simulink model "BallPlate_FLControl"  (R2018b)
settings: Solver=FixedStepAuto  StartTime=0.0  StopTime=20  FixedStep=0.01  RelTol=1e-5
undefined symbols (not defined in the file or in its folder): K
libraries: vrlib x42, simulink x5, aerolibanimutils x3, powerlib_meascontrol x1
(part 2 of 2)

== system BallPlate_FLControl/Feedback linearized 3/Subsystem ==
  tau : Inport
  Ball and Plate dynamic : MATLAB Function  TreatAsAtomicUnit=on
  Constant : Constant  Value=[0.0001;0.0001;.0001;.0001]
  Constant1 : Constant  Value=[.0001;.0001;.0001;.0001]
  Integrator : Integrator  InitialConditionSource=external  InitialCondition=[0;0;0;0]
  Integrator1 : Integrator  InitialConditionSource=external  InitialCondition=[0; 0; 0; 0]
  q : Outport
  dq : Outport  Port=2
  wires:
  tau/1 -> Ball and Plate dynamic/1(tau)
  Integrator1/1 -> q/1, Ball and Plate dynamic/2(q)
  Integrator/1 -> dq/1, Integrator1/1, Ball and Plate dynamic/3(dq)
  Ball and Plate dynamic/1(ddq) -> Integrator/1
  Constant/1 -> Integrator/2
  Constant1/1 -> Integrator1/2

== system BallPlate_FLControl/Feedback linearized 4/Feedback Linearization ==
  nu : Inport
  q : Inport  Port=2
  dq : Inport  Port=3
  Einv_matrix : MATLAB Function  TreatAsAtomicUnit=on
  Gamma_matrix : MATLAB Function  TreatAsAtomicUnit=on
  Matrix Multiply : Product  Multiplication=Matrix(*)
  Matrix Multiply1 : Product  Multiplication=Matrix(*)
  Sum : Sum  Inputs=+-
  u : Outport
  wires:
  Sum/1 -> u/1
  Matrix Multiply1/1 -> Sum/2
  Matrix Multiply/1 -> Sum/1
  Gamma_matrix/1(Gamma) -> Matrix Multiply1/2
  nu/1 -> Matrix Multiply/2
  Einv_matrix/1(Einv) -> Matrix Multiply/1, Matrix Multiply1/1
  dq/1 -> Einv_matrix/2(dq), Gamma_matrix/2(dq)
  q/1 -> Einv_matrix/1(q), Gamma_matrix/1(q)

== system BallPlate_FLControl/Feedback linearized 4/Subsystem ==
  tau : Inport
  Ball and Plate dynamic : MATLAB Function  TreatAsAtomicUnit=on
  Constant : Constant  Value=[0.0001;0.0001;.0001;.0001]
  Constant1 : Constant  Value=[.0001;.0001;.0001;.0001]
  Integrator : Integrator  InitialConditionSource=external  InitialCondition=[0;0;0;0]
  Integrator1 : Integrator  InitialConditionSource=external  InitialCondition=[0; 0; 0; 0]
  q : Outport
  dq : Outport  Port=2
  wires:
  Constant1/1 -> Integrator1/2
  Constant/1 -> Integrator/2
  Ball and Plate dynamic/1(ddq) -> Integrator/1
  Integrator/1 -> Ball and Plate dynamic/3(dq), Integrator1/1, dq/1
  Integrator1/1 -> Ball and Plate dynamic/2(q), q/1
  tau/1 -> Ball and Plate dynamic/1(tau)

== system BallPlate_FLControl/Feedback linearized 5/Feedback Linearization ==
  nu : Inport
  q : Inport  Port=2
  dq : Inport  Port=3
  Einv_matrix : MATLAB Function  TreatAsAtomicUnit=on
  Gamma_matrix : MATLAB Function  TreatAsAtomicUnit=on
  Matrix Multiply : Product  Multiplication=Matrix(*)
  Matrix Multiply1 : Product  Multiplication=Matrix(*)
  Sum : Sum  Inputs=+-
  u : Outport
  wires:
  q/1 -> Gamma_matrix/1(q), Einv_matrix/1(q)
  dq/1 -> Gamma_matrix/2(dq), Einv_matrix/2(dq)
  Einv_matrix/1(Einv) -> Matrix Multiply1/1, Matrix Multiply/1
  nu/1 -> Matrix Multiply/2
  Gamma_matrix/1(Gamma) -> Matrix Multiply1/2
  Matrix Multiply/1 -> Sum/1
  Matrix Multiply1/1 -> Sum/2
  Sum/1 -> u/1

== system BallPlate_FLControl/Feedback linearized 5/Subsystem ==
  tau : Inport
  Ball and Plate dynamic : MATLAB Function  TreatAsAtomicUnit=on
  Constant : Constant  Value=[0.0001;0.0001;.0001;.0001]
  Constant1 : Constant  Value=[.0001;.0001;.0001;.0001]
  Integrator : Integrator  InitialConditionSource=external  InitialCondition=[0;0;0;0]
  Integrator1 : Integrator  InitialConditionSource=external  InitialCondition=[0; 0; 0; 0]
  q : Outport
  dq : Outport  Port=2
  wires:
  tau/1 -> Ball and Plate dynamic/1(tau)
  Integrator1/1 -> q/1, Ball and Plate dynamic/2(q)
  Integrator/1 -> dq/1, Integrator1/1, Ball and Plate dynamic/3(dq)
  Ball and Plate dynamic/1(ddq) -> Integrator/1
  Constant/1 -> Integrator/2
  Constant1/1 -> Integrator1/2

== system BallPlate_FLControl/Visualization parsing1/Rotation composition 1 ==
  alpha : Inport
  beta : Inport  Port=2
  Rotation : MATLAB Function  TreatAsAtomicUnit=on
  Rotation Matrix to VRML Rotation : vrlib/Utilities/Rotation Matrix to VRML Rotation  maxzero=1e-12
      settings: SourceProductName=Simulink 3D Animation  SourceProductBaseCode=VR
  Axis/angle : Outport
  wires:
  alpha/1 -> Rotation/1(alpha)
  Rotation Matrix to VRML Rotation/1 -> Axis/angle/1
  beta/1 -> Rotation/2(beta)
  Rotation/1(R) -> Rotation Matrix to VRML Rotation/1

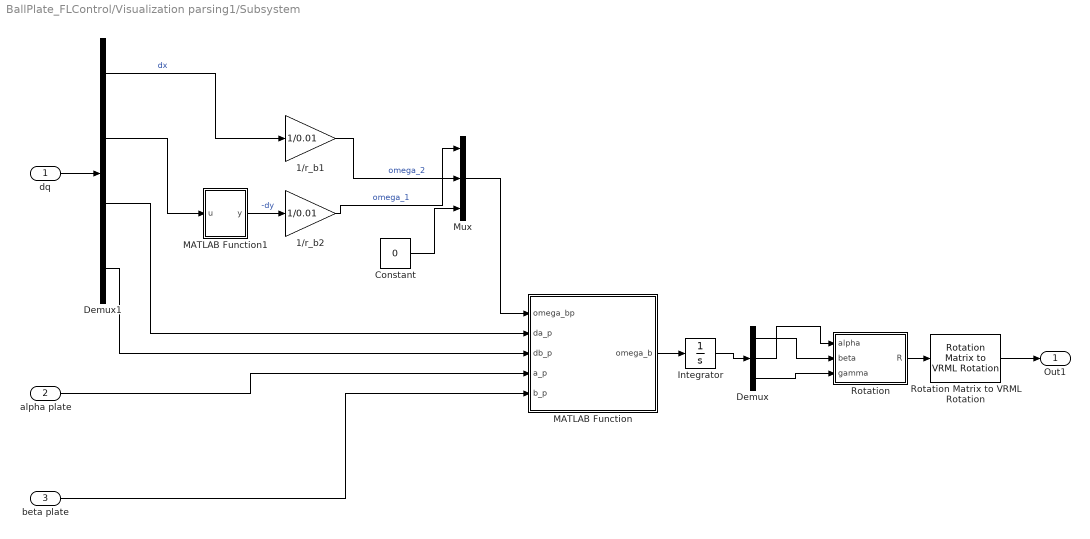
== system BallPlate_FLControl/Visualization parsing1/Subsystem ==
  dq : Inport
  alpha plate : Inport  Port=2
  beta plate : Inport  Port=3
  1/r_b1 : Gain  Gain=1/0.01
  1/r_b2 : Gain  Gain=1/0.01
  Constant : Constant  Value=0
  Demux : Demux  Outputs=3
  Demux1 : Demux
  Integrator : Integrator
  MATLAB Function : MATLAB Function  TreatAsAtomicUnit=on
  MATLAB Function1 : MATLAB Function  TreatAsAtomicUnit=on
  Mux : Mux  Inputs=3
  Rotation : MATLAB Function  TreatAsAtomicUnit=on
  Rotation Matrix to VRML Rotation : vrlib/Utilities/Rotation Matrix to VRML Rotation  maxzero=1e-12
      settings: SourceProductName=Simulink 3D Animation  SourceProductBaseCode=VR
  Out1 : Outport
  wires:
  MATLAB Function1/1(y) -> 1/r_b2/1  "-dy"
  Demux1/4 -> MATLAB Function/3(db_p)
  Demux1/3 -> MATLAB Function/2(da_p)
  Demux1/1 -> 1/r_b1/1  "dx"
  Demux1/2 -> MATLAB Function1/1(u)
  Rotation Matrix to VRML Rotation/1 -> Out1/1
  dq/1 -> Demux1/1
  Demux/1 -> Rotation/2(beta)
  alpha plate/1 -> MATLAB Function/4(a_p)
  beta plate/1 -> MATLAB Function/5(b_p)
  1/r_b1/1 -> Mux/2  "omega_2"
  1/r_b2/1 -> Mux/1  "omega_1"
  Mux/1 -> MATLAB Function/1(omega_bp)
  MATLAB Function/1(omega_b) -> Integrator/1
  Integrator/1 -> Demux/1
  Rotation/1(R) -> Rotation Matrix to VRML Rotation/1
  Demux/2 -> Rotation/1(alpha)
  Demux/3 -> Rotation/3(gamma)
  Constant/1 -> Mux/3

== system BallPlate_FLControl/Visualization parsing2/Rotation composition 1 ==
  alpha : Inport
  beta : Inport  Port=2
  Rotation : MATLAB Function  TreatAsAtomicUnit=on
  Rotation Matrix to VRML Rotation : vrlib/Utilities/Rotation Matrix to VRML Rotation  maxzero=1e-12
      settings: SourceProductName=Simulink 3D Animation  SourceProductBaseCode=VR
  Axis/angle : Outport
  wires:
  alpha/1 -> Rotation/1(alpha)
  Rotation Matrix to VRML Rotation/1 -> Axis/angle/1
  beta/1 -> Rotation/2(beta)
  Rotation/1(R) -> Rotation Matrix to VRML Rotation/1

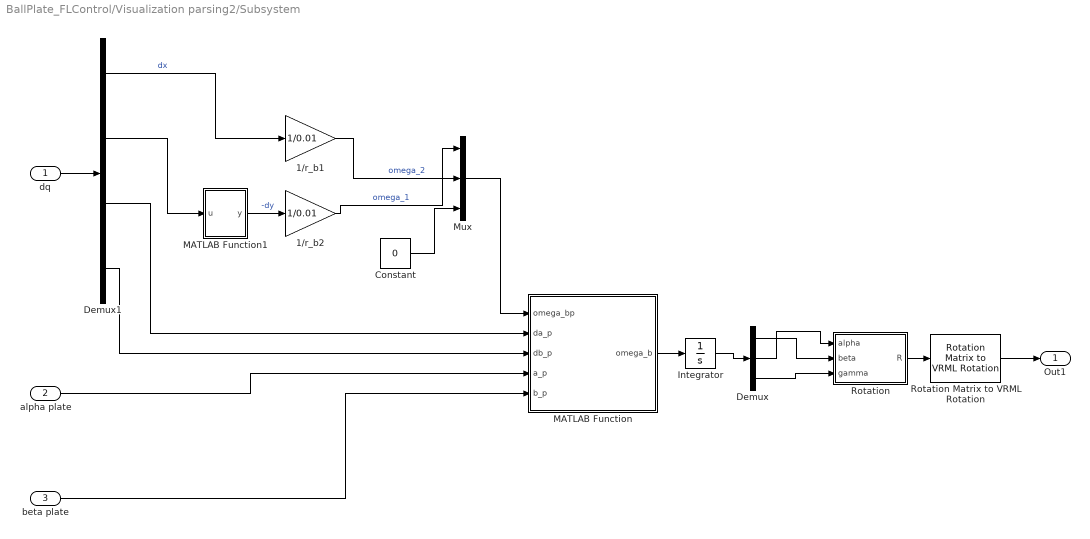
== system BallPlate_FLControl/Visualization parsing2/Subsystem ==
  dq : Inport
  alpha plate : Inport  Port=2
  beta plate : Inport  Port=3
  1/r_b1 : Gain  Gain=1/0.01
  1/r_b2 : Gain  Gain=1/0.01
  Constant : Constant  Value=0
  Demux : Demux  Outputs=3
  Demux1 : Demux
  Integrator : Integrator
  MATLAB Function : MATLAB Function  TreatAsAtomicUnit=on
  MATLAB Function1 : MATLAB Function  TreatAsAtomicUnit=on
  Mux : Mux  Inputs=3
  Rotation : MATLAB Function  TreatAsAtomicUnit=on
  Rotation Matrix to VRML Rotation : vrlib/Utilities/Rotation Matrix to VRML Rotation  maxzero=1e-12
      settings: SourceProductName=Simulink 3D Animation  SourceProductBaseCode=VR
  Out1 : Outport
  wires:
  MATLAB Function1/1(y) -> 1/r_b2/1  "-dy"
  Demux1/4 -> MATLAB Function/3(db_p)
  Demux1/3 -> MATLAB Function/2(da_p)
  Demux1/1 -> 1/r_b1/1  "dx"
  Demux1/2 -> MATLAB Function1/1(u)
  Rotation Matrix to VRML Rotation/1 -> Out1/1
  dq/1 -> Demux1/1
  Demux/1 -> Rotation/2(beta)
  alpha plate/1 -> MATLAB Function/4(a_p)
  beta plate/1 -> MATLAB Function/5(b_p)
  1/r_b1/1 -> Mux/2  "omega_2"
  1/r_b2/1 -> Mux/1  "omega_1"
  Mux/1 -> MATLAB Function/1(omega_bp)
  MATLAB Function/1(omega_b) -> Integrator/1
  Integrator/1 -> Demux/1
  Rotation/1(R) -> Rotation Matrix to VRML Rotation/1
  Demux/2 -> Rotation/1(alpha)
  Demux/3 -> Rotation/3(gamma)
  Constant/1 -> Mux/3

== system BallPlate_FLControl/Visualization parsing3/Rotation composition ==
  omega_b : Inport
  Demux : Demux  Outputs=2
  Integrator : Integrator  InitialCondition=[0; 0]
  Rotation : MATLAB Function  TreatAsAtomicUnit=on
  Rotation Matrix to VRML Rotation : vrlib/Utilities/Rotation Matrix to VRML Rotation  maxzero=1e-12
      settings: SourceProductName=Simulink 3D Animation  SourceProductBaseCode=VR
  Axis/angle : Outport
  wires:
  omega_b/1 -> Integrator/1
  Integrator/1 -> Demux/1
  Rotation Matrix to VRML Rotation/1 -> Axis/angle/1
  Rotation/1(R) -> Rotation Matrix to VRML Rotation/1
  Demux/1 -> Rotation/1(alpha)
  Demux/2 -> Rotation/2(beta)

== system BallPlate_FLControl/Visualization parsing3/Rotation composition 1 ==
  alpha : Inport
  beta : Inport  Port=2
  Rotation : MATLAB Function  TreatAsAtomicUnit=on
  Rotation Matrix to VRML Rotation : vrlib/Utilities/Rotation Matrix to VRML Rotation  maxzero=1e-12
      settings: SourceProductName=Simulink 3D Animation  SourceProductBaseCode=VR
  Axis/angle : Outport
  wires:
  alpha/1 -> Rotation/1(alpha)
  Rotation Matrix to VRML Rotation/1 -> Axis/angle/1
  beta/1 -> Rotation/2(beta)
  Rotation/1(R) -> Rotation Matrix to VRML Rotation/1

== system BallPlate_FLControl/Visualization parsing4/Rotation composition ==
  omega_b : Inport
  Demux : Demux  Outputs=2
  Integrator : Integrator  InitialCondition=[0; 0]
  Rotation : MATLAB Function  TreatAsAtomicUnit=on
  Rotation Matrix to VRML Rotation : vrlib/Utilities/Rotation Matrix to VRML Rotation  maxzero=1e-12
      settings: SourceProductName=Simulink 3D Animation  SourceProductBaseCode=VR
  Axis/angle : Outport
  wires:
  Demux/2 -> Rotation/2(beta)
  Demux/1 -> Rotation/1(alpha)
  Rotation/1(R) -> Rotation Matrix to VRML Rotation/1
  Rotation Matrix to VRML Rotation/1 -> Axis/angle/1
  Integrator/1 -> Demux/1
  omega_b/1 -> Integrator/1

== system BallPlate_FLControl/Visualization parsing4/Rotation composition 1 ==
  alpha : Inport
  beta : Inport  Port=2
  Rotation : MATLAB Function  TreatAsAtomicUnit=on
  Rotation Matrix to VRML Rotation : vrlib/Utilities/Rotation Matrix to VRML Rotation  maxzero=1e-12
      settings: SourceProductName=Simulink 3D Animation  SourceProductBaseCode=VR
  Axis/angle : Outport
  wires:
  Rotation/1(R) -> Rotation Matrix to VRML Rotation/1
  beta/1 -> Rotation/2(beta)
  Rotation Matrix to VRML Rotation/1 -> Axis/angle/1
  alpha/1 -> Rotation/1(alpha)

== system BallPlate_FLControl/Visualization parsing5/Rotation composition ==
  omega_b : Inport
  Demux : Demux  Outputs=2
  Integrator : Integrator  InitialCondition=[0; 0]
  Rotation : MATLAB Function  TreatAsAtomicUnit=on
  Rotation Matrix to VRML Rotation : vrlib/Utilities/Rotation Matrix to VRML Rotation  maxzero=1e-12
      settings: SourceProductName=Simulink 3D Animation  SourceProductBaseCode=VR
  Axis/angle : Outport
  wires:
  omega_b/1 -> Integrator/1
  Integrator/1 -> Demux/1
  Rotation Matrix to VRML Rotation/1 -> Axis/angle/1
  Rotation/1(R) -> Rotation Matrix to VRML Rotation/1
  Demux/1 -> Rotation/1(alpha)
  Demux/2 -> Rotation/2(beta)

== system BallPlate_FLControl/Visualization parsing5/Rotation composition 1 ==
  alpha : Inport
  beta : Inport  Port=2
  Rotation : MATLAB Function  TreatAsAtomicUnit=on
  Rotation Matrix to VRML Rotation : vrlib/Utilities/Rotation Matrix to VRML Rotation  maxzero=1e-12
      settings: SourceProductName=Simulink 3D Animation  SourceProductBaseCode=VR
  Axis/angle : Outport
  wires:
  alpha/1 -> Rotation/1(alpha)
  Rotation Matrix to VRML Rotation/1 -> Axis/angle/1
  beta/1 -> Rotation/2(beta)
  Rotation/1(R) -> Rotation Matrix to VRML Rotation/1

== system BallPlate_FLControl/Visualization parsing6/Rotation composition ==
  omega_b : Inport
  Demux : Demux  Outputs=2
  Integrator : Integrator  InitialCondition=[0; 0]
  Rotation : MATLAB Function  TreatAsAtomicUnit=on
  Rotation Matrix to VRML Rotation : vrlib/Utilities/Rotation Matrix to VRML Rotation  maxzero=1e-12
      settings: SourceProductName=Simulink 3D Animation  SourceProductBaseCode=VR
  Axis/angle : Outport
  wires:
  omega_b/1 -> Integrator/1
  Integrator/1 -> Demux/1
  Rotation Matrix to VRML Rotation/1 -> Axis/angle/1
  Rotation/1(R) -> Rotation Matrix to VRML Rotation/1
  Demux/1 -> Rotation/1(alpha)
  Demux/2 -> Rotation/2(beta)

== system BallPlate_FLControl/Visualization parsing6/Rotation composition 1 ==
  alpha : Inport
  beta : Inport  Port=2
  Rotation : MATLAB Function  TreatAsAtomicUnit=on
  Rotation Matrix to VRML Rotation : vrlib/Utilities/Rotation Matrix to VRML Rotation  maxzero=1e-12
      settings: SourceProductName=Simulink 3D Animation  SourceProductBaseCode=VR
  Axis/angle : Outport
  wires:
  alpha/1 -> Rotation/1(alpha)
  Rotation Matrix to VRML Rotation/1 -> Axis/angle/1
  beta/1 -> Rotation/2(beta)
  Rotation/1(R) -> Rotation Matrix to VRML Rotation/1

== system BallPlate_FLControl/Visualization parsing7/Rotation composition ==
  omega_b : Inport
  Demux : Demux  Outputs=2
  Integrator : Integrator  InitialCondition=[0; 0]
  Rotation : MATLAB Function  TreatAsAtomicUnit=on
  Rotation Matrix to VRML Rotation : vrlib/Utilities/Rotation Matrix to VRML Rotation  maxzero=1e-12
      settings: SourceProductName=Simulink 3D Animation  SourceProductBaseCode=VR
  Axis/angle : Outport
  wires:
  Demux/2 -> Rotation/2(beta)
  Demux/1 -> Rotation/1(alpha)
  Rotation/1(R) -> Rotation Matrix to VRML Rotation/1
  Rotation Matrix to VRML Rotation/1 -> Axis/angle/1
  Integrator/1 -> Demux/1
  omega_b/1 -> Integrator/1

== system BallPlate_FLControl/Visualization parsing7/Rotation composition 1 ==
  alpha : Inport
  beta : Inport  Port=2
  Rotation : MATLAB Function  TreatAsAtomicUnit=on
  Rotation Matrix to VRML Rotation : vrlib/Utilities/Rotation Matrix to VRML Rotation  maxzero=1e-12
      settings: SourceProductName=Simulink 3D Animation  SourceProductBaseCode=VR
  Axis/angle : Outport
  wires:
  Rotation/1(R) -> Rotation Matrix to VRML Rotation/1
  beta/1 -> Rotation/2(beta)
  Rotation Matrix to VRML Rotation/1 -> Axis/angle/1
  alpha/1 -> Rotation/1(alpha)

== matlab function BallPlate_FLControl/Visualization parsing1/MATLAB Function1 ==
  data: u input; y output
function y = fcn(u)

y = -u;

== matlab function BallPlate_FLControl/Feedback linearized /Subsystem/Ball and Plate dynamic ==
  data: tau input; ddq output; q input; dq input
function ddq = InvDyn_BP(tau, q, dq)

if size(dq,2) == 3
    dq = dq';
end

tau1 = [0; 0; tau(1); tau(2)];

% B, C, G matrices
[B, C, G] = BCG_BP(q, dq);

% Inverse dynamic
ddq = B\(tau1 - C*dq - G); 

end

== matlab function BallPlate_FLControl/Feedback linearized 1/Coordinate transform ==
  data: q input; z output; dq input
function z = fcn(q,dq)

    [m_b, r_b, I_b, ~, ~] = Parameters_BP;

    x1 = q(1);
    x2 = q(2);
    x3 = q(3);
    x4 = q(4);
    x5 = dq(1);
    x6 = dq(2);
    x7 = dq(3);
    x8 = dq(4);

    B1 = m_b/(I_b/r_b^2 + m_b);
    g = 9.81;



    z = [x1;
         x5;
         B1*(x1*x7^2 - g*sin(x3));
         B1*x5*x7^2 - B1*g*cos(x3)*x7;
         x2;
         x6;
         B1*(x2*x8^2 - g*sin(x4));
         B1*x6*x8^2 - B1*g*cos(x4)*x8];

== matlab function BallPlate_FLControl/Feedback linearized /Feedback Linearization/Einv_matrix ==
  data: q input; Einv output; dq input
function Einv = fcn(q,dq)

[m_b, r_b, I_b, ~, ~] = Parameters_BP;

x3 = q(3);
x4 = q(4);
x5 = dq(1);
x6 = dq(2);
x7 = dq(3);
x8 = dq(4);

B1 = m_b/(I_b/r_b^2 + m_b);
g = 9.81;

% E = [jacobian(dddy1,x)*g1; jacobian(dddy1,x)*g2;
%      jacobian(dddy2,x)*g1; jacobian(dddy2,x)*g2];

E11 = (2*B1*x5*x7 - B1*g*cos(x3));
E22 = (2*B1*x6*x8 - B1*g*cos(x4));

E = diag([E11, E22]);

Einv = inv(E);

== matlab function BallPlate_FLControl/Feedback linearized 1/Feedback Linearization/Einv_matrix ==
  data: q input; Einv output; dq input
function Einv = fcn(q,dq)

[m_b, r_b, I_b, ~, ~] = Parameters_BP;

x3 = q(3);
x4 = q(4);
x5 = dq(1);
x6 = dq(2);
x7 = dq(3);
x8 = dq(4);

B1 = m_b/(I_b/r_b^2 + m_b);
g = 9.81;

% E = [jacobian(dddy1,x)*g1; jacobian(dddy1,x)*g2;
%      jacobian(dddy2,x)*g1; jacobian(dddy2,x)*g2];

E11 = (2*B1*x5*x7 - B1*g*cos(x3));
E22 = (2*B1*x6*x8 - B1*g*cos(x4));

E = diag([E11, E22]);

Einv = inv(E);

== matlab function BallPlate_FLControl/Visualization parsing1/Rotation ==
  data: alpha input; R output; beta input
function R = fcn(alpha, beta)

    Rx = [1 0 0; 0 cos(beta) -sin(beta); 0 sin(beta) cos(beta)];
    Ry = [cos(alpha) 0 sin(alpha); 0 1 0; -sin(alpha) 0 cos(alpha)];

R = Rx*Ry;

== matlab function BallPlate_FLControl/Feedback linearized /Feedback Linearization/Gamma_matrix ==
  data: q input; Gamma output; dq input
function Gamma = fcn(q,dq)

[m_b, r_b, I_b, ~, ~] = Parameters_BP;

x1 = q(1);
x2 = q(2);
x3 = q(3);
x4 = q(4);
x7 = dq(3);
x8 = dq(4);

B1 = m_b/(I_b/r_b^2 + m_b);
g = 9.81;

% Gamma = jacobian(dddy1,x)*f1;
%         jacobian(dddy2,x)*f1];

Gamma1 = B1^2*x7^2*(x1*x7^2 - g*sin(x3)) + B1*g*x7^2*sin(x3);
Gamma2 = B1^2*x8^2*(x2*x8^2 - g*sin(x4)) + B1*g*x8^2*sin(x4);

Gamma = [Gamma1; Gamma2];

== matlab function BallPlate_FLControl/Feedback linearized /Coordinate transform ==
  data: q input; z output; dq input
function z = fcn(q,dq)

    [m_b, r_b, I_b, ~, ~] = Parameters_BP;

    x1 = q(1);
    x2 = q(2);
    x3 = q(3);
    x4 = q(4);
    x5 = dq(1);
    x6 = dq(2);
    x7 = dq(3);
    x8 = dq(4);

    B1 = m_b/(I_b/r_b^2 + m_b);
    g = 9.81;



    z = [x1;
         x5;
         B1*(x1*x7^2 - g*sin(x3));
         B1*x5*x7^2 - B1*g*cos(x3)*x7;
         x2;
         x6;
         B1*(x2*x8^2 - g*sin(x4));
         B1*x6*x8^2 - B1*g*cos(x4)*x8];

== matlab function BallPlate_FLControl/Feedback linearized 1/Feedback Linearization/Gamma_matrix ==
  data: q input; Gamma output; dq input
function Gamma = fcn(q,dq)

[m_b, r_b, I_b, ~, ~] = Parameters_BP;

x1 = q(1);
x2 = q(2);
x3 = q(3);
x4 = q(4);
x7 = dq(3);
x8 = dq(4);

B1 = m_b/(I_b/r_b^2 + m_b);
g = 9.81;

% Gamma = jacobian(dddy1,x)*f1;
%         jacobian(dddy2,x)*f1];

Gamma1 = B1^2*x7^2*(x1*x7^2 - g*sin(x3)) + B1*g*x7^2*sin(x3);
Gamma2 = B1^2*x8^2*(x2*x8^2 - g*sin(x4)) + B1*g*x8^2*sin(x4);

Gamma = [Gamma1; Gamma2];

== matlab function BallPlate_FLControl/Subsystem1/Ball and Plate dynamic ==
  data: tau input; ddq output; q input; dq input
function ddq = InvDyn_BP(tau, q, dq)

if size(dq,2) == 3
    dq = dq';
end

tau1 = [0; 0; tau(1); tau(2)];

% B, C, G matrices
[B, C, G] = BCG_BP(q, dq);

% Inverse dynamic
ddq = B\(tau1 - C*dq - G); 

end

== matlab function BallPlate_FLControl/Visualization parsing1/Rotation composition 1/Rotation ==
  data: alpha input; R output; beta input
function R = fcn(alpha, beta)
    
    Rx = [1 0 0; 0 cos(beta) -sin(beta); 0 sin(beta) cos(beta)];
    Ry = [cos(alpha) 0 sin(alpha); 0 1 0; -sin(alpha) 0 cos(alpha)];

R = Rx*Ry;

== matlab function BallPlate_FLControl/Visualization parsing1/Subsystem/MATLAB Function ==
  data: omega_bp input; da_p input; db_p input; omega_b output; a_p input; b_p input
function omega_b = fcn(omega_bp, da_p, db_p, a_p, b_p)

omega_p = [da_p*cos(b_p); db_p; da_p*sin(b_p)];

omega_b = omega_bp + omega_p;

== matlab function BallPlate_FLControl/Visualization parsing1/Subsystem/MATLAB Function1 ==
  data: u input; y output
function y = fcn(u)

y = -u;

== matlab function BallPlate_FLControl/Visualization parsing1/Subsystem/Rotation ==
  data: alpha input; R output; beta input; gamma input
function R = fcn(alpha, beta, gamma)
    
    Rx = [1 0 0; 0 cos(beta) -sin(beta); 0 sin(beta) cos(beta)];
    Ry = [cos(alpha) 0 sin(alpha); 0 1 0; -sin(alpha) 0 cos(alpha)];
    Rz = [cos(gamma) -sin(gamma) 0; sin(gamma) cos(gamma) 0; 0 0 1];

    
R = Rx*Ry*Rz;

== matlab function BallPlate_FLControl/Feedback linearized 1/Subsystem/Ball and Plate dynamic ==
  data: tau input; ddq output; q input; dq input
function ddq = InvDyn_BP(tau, q, dq)

if size(dq,2) == 3
    dq = dq';
end

tau1 = [0; 0; tau(1); tau(2)];

% B, C, G matrices
[B, C, G] = BCG_BP(q, dq);

% Inverse dynamic
ddq = B\(tau1 - C*dq - G); 

end

== matlab function BallPlate_FLControl/Subsystem2/Ball and Plate dynamic ==
  data: tau input; ddq output; q input; dq input
function ddq = InvDyn_BP(tau, q, dq)

if size(dq,2) == 3
    dq = dq';
end

tau1 = [0; 0; tau(1); tau(2)];

% B, C, G matrices
[B, C, G] = BCG_BP(q, dq);

% Inverse dynamic
ddq = B\(tau1 - C*dq - G); 

end

== matlab function BallPlate_FLControl/Visualization parsing2/Rotation ==
  data: alpha input; R output; beta input
function R = fcn(alpha, beta)

    Rx = [1 0 0; 0 cos(beta) -sin(beta); 0 sin(beta) cos(beta)];
    Ry = [cos(alpha) 0 sin(alpha); 0 1 0; -sin(alpha) 0 cos(alpha)];

R = Rx*Ry;

== matlab function BallPlate_FLControl/Visualization parsing2/Rotation composition 1/Rotation ==
  data: alpha input; R output; beta input
function R = fcn(alpha, beta)
    
    Rx = [1 0 0; 0 cos(beta) -sin(beta); 0 sin(beta) cos(beta)];
    Ry = [cos(alpha) 0 sin(alpha); 0 1 0; -sin(alpha) 0 cos(alpha)];

R = Rx*Ry;

== matlab function BallPlate_FLControl/Visualization parsing2/Subsystem/MATLAB Function ==
  data: omega_bp input; da_p input; db_p input; omega_b output; a_p input; b_p input
function omega_b = fcn(omega_bp, da_p, db_p, a_p, b_p)

omega_p = [da_p*cos(b_p); db_p; da_p*sin(b_p)];

omega_b = omega_bp + omega_p;

== matlab function BallPlate_FLControl/Visualization parsing2/Subsystem/MATLAB Function1 ==
  data: u input; y output
function y = fcn(u)

y = -u;

== matlab function BallPlate_FLControl/Visualization parsing2/Subsystem/Rotation ==
  data: alpha input; R output; beta input; gamma input
function R = fcn(alpha, beta, gamma)
    
    Rx = [1 0 0; 0 cos(beta) -sin(beta); 0 sin(beta) cos(beta)];
    Ry = [cos(alpha) 0 sin(alpha); 0 1 0; -sin(alpha) 0 cos(alpha)];
    Rz = [cos(gamma) -sin(gamma) 0; sin(gamma) cos(gamma) 0; 0 0 1];

    
R = Rx*Ry*Rz;

== matlab function BallPlate_FLControl/Visualization parsing3/MATLAB Function ==
  data: u input; y output
function y = fcn(u)

y = -u;

== matlab function BallPlate_FLControl/Visualization parsing3/Rotation ==
  data: alpha input; R output; beta input
function R = fcn(alpha, beta)

    Rx = [1 0 0; 0 cos(beta) -sin(beta); 0 sin(beta) cos(beta)];
    Ry = [cos(alpha) 0 sin(alpha); 0 1 0; -sin(alpha) 0 cos(alpha)];

R = Rx*Ry;

== matlab function BallPlate_FLControl/Visualization parsing3/Rotation composition/Rotation ==
  data: alpha input; R output; beta input
function R = fcn(alpha, beta)

    alpha = -alpha;
    beta = -beta;
    Rx = [1 0 0; 0 cos(beta) -sin(beta); 0 sin(beta) cos(beta)];
    Ry = [cos(alpha) 0 sin(alpha); 0 1 0; -sin(alpha) 0 cos(alpha)];

R = Rx*Ry;

== matlab function BallPlate_FLControl/Visualization parsing3/Rotation composition 1/Rotation ==
  data: alpha input; R output; beta input
function R = fcn(alpha, beta)
    
    Rx = [1 0 0; 0 cos(beta) -sin(beta); 0 sin(beta) cos(beta)];
    Ry = [cos(alpha) 0 sin(alpha); 0 1 0; -sin(alpha) 0 cos(alpha)];

R = Rx*Ry;

== matlab function BallPlate_FLControl/Visualization parsing4/MATLAB Function ==
  data: u input; y output
function y = fcn(u)

y = -u;

== matlab function BallPlate_FLControl/Visualization parsing4/Rotation ==
  data: alpha input; R output; beta input
function R = fcn(alpha, beta)

    Rx = [1 0 0; 0 cos(beta) -sin(beta); 0 sin(beta) cos(beta)];
    Ry = [cos(alpha) 0 sin(alpha); 0 1 0; -sin(alpha) 0 cos(alpha)];

R = Rx*Ry;

== matlab function BallPlate_FLControl/Visualization parsing4/Rotation composition/Rotation ==
  data: alpha input; R output; beta input
function R = fcn(alpha, beta)

    alpha = -alpha;
    beta = -beta;
    Rx = [1 0 0; 0 cos(beta) -sin(beta); 0 sin(beta) cos(beta)];
    Ry = [cos(alpha) 0 sin(alpha); 0 1 0; -sin(alpha) 0 cos(alpha)];

R = Rx*Ry;

== matlab function BallPlate_FLControl/Visualization parsing4/Rotation composition 1/Rotation ==
  data: alpha input; R output; beta input
function R = fcn(alpha, beta)
    
    Rx = [1 0 0; 0 cos(beta) -sin(beta); 0 sin(beta) cos(beta)];
    Ry = [cos(alpha) 0 sin(alpha); 0 1 0; -sin(alpha) 0 cos(alpha)];

R = Rx*Ry;

== matlab function BallPlate_FLControl/Feedback linearized 2/Coordinate transform ==
  data: q input; z output; dq input
function z = fcn(q,dq)

    [m_b, r_b, I_b, ~, ~] = Parameters_BP;

    x1 = q(1);
    x2 = q(2);
    x3 = q(3);
    x4 = q(4);
    x5 = dq(1);
    x6 = dq(2);
    x7 = dq(3);
    x8 = dq(4);

    B1 = m_b/(I_b/r_b^2 + m_b);
    g = 9.81;



    z = [x1;
         x5;
         B1*(x1*x7^2 - g*sin(x3));
         B1*x5*x7^2 - B1*g*cos(x3)*x7;
         x2;
         x6;
         B1*(x2*x8^2 - g*sin(x4));
         B1*x6*x8^2 - B1*g*cos(x4)*x8];

== matlab function BallPlate_FLControl/Feedback linearized 2/Feedback Linearization/Einv_matrix ==
  data: q input; Einv output; dq input
function Einv = fcn(q,dq)

[m_b, r_b, I_b, ~, ~] = Parameters_BP;

x3 = q(3);
x4 = q(4);
x5 = dq(1);
x6 = dq(2);
x7 = dq(3);
x8 = dq(4);

B1 = m_b/(I_b/r_b^2 + m_b);
g = 9.81;

% E = [jacobian(dddy1,x)*g1; jacobian(dddy1,x)*g2;
%      jacobian(dddy2,x)*g1; jacobian(dddy2,x)*g2];

E11 = (2*B1*x5*x7 - B1*g*cos(x3));
E22 = (2*B1*x6*x8 - B1*g*cos(x4));

E = diag([E11, E22]);

Einv = inv(E);

== matlab function BallPlate_FLControl/Feedback linearized 2/Feedback Linearization/Gamma_matrix ==
  data: q input; Gamma output; dq input
function Gamma = fcn(q,dq)

[m_b, r_b, I_b, ~, ~] = Parameters_BP;

x1 = q(1);
x2 = q(2);
x3 = q(3);
x4 = q(4);
x7 = dq(3);
x8 = dq(4);

B1 = m_b/(I_b/r_b^2 + m_b);
g = 9.81;

% Gamma = jacobian(dddy1,x)*f1;
%         jacobian(dddy2,x)*f1];

Gamma1 = B1^2*x7^2*(x1*x7^2 - g*sin(x3)) + B1*g*x7^2*sin(x3);
Gamma2 = B1^2*x8^2*(x2*x8^2 - g*sin(x4)) + B1*g*x8^2*sin(x4);

Gamma = [Gamma1; Gamma2];

== matlab function BallPlate_FLControl/Feedback linearized 2/Subsystem/Ball and Plate dynamic ==
  data: tau input; ddq output; q input; dq input
function ddq = InvDyn_BP(tau, q, dq)

if size(dq,2) == 3
    dq = dq';
end

tau1 = [0; 0; tau(1); tau(2)];

% B, C, G matrices
[B, C, G] = BCG_BP(q, dq);

% Inverse dynamic
ddq = B\(tau1 - C*dq - G); 

end

== matlab function BallPlate_FLControl/Visualization parsing5/MATLAB Function ==
  data: u input; y output
function y = fcn(u)

y = -u;

== matlab function BallPlate_FLControl/Visualization parsing5/Rotation ==
  data: alpha input; R output; beta input
function R = fcn(alpha, beta)

    Rx = [1 0 0; 0 cos(beta) -sin(beta); 0 sin(beta) cos(beta)];
    Ry = [cos(alpha) 0 sin(alpha); 0 1 0; -sin(alpha) 0 cos(alpha)];

R = Rx*Ry;

== matlab function BallPlate_FLControl/Visualization parsing5/Rotation composition/Rotation ==
  data: alpha input; R output; beta input
function R = fcn(alpha, beta)

    alpha = -alpha;
    beta = -beta;
    Rx = [1 0 0; 0 cos(beta) -sin(beta); 0 sin(beta) cos(beta)];
    Ry = [cos(alpha) 0 sin(alpha); 0 1 0; -sin(alpha) 0 cos(alpha)];

R = Rx*Ry;

== matlab function BallPlate_FLControl/Visualization parsing5/Rotation composition 1/Rotation ==
  data: alpha input; R output; beta input
function R = fcn(alpha, beta)
    
    Rx = [1 0 0; 0 cos(beta) -sin(beta); 0 sin(beta) cos(beta)];
    Ry = [cos(alpha) 0 sin(alpha); 0 1 0; -sin(alpha) 0 cos(alpha)];

R = Rx*Ry;

== matlab function BallPlate_FLControl/Feedback linearized 3/Coordinate transform ==
  data: q input; z output; dq input
function z = fcn(q,dq)

    [m_b, r_b, I_b, ~, ~] = Parameters_BP;

    x1 = q(1);
    x2 = q(2);
    x3 = q(3);
    x4 = q(4);
    x5 = dq(1);
    x6 = dq(2);
    x7 = dq(3);
    x8 = dq(4);

    B1 = m_b/(I_b/r_b^2 + m_b);
    g = 9.81;



    z = [x1;
         x5;
         B1*(x1*x7^2 - g*sin(x3));
         B1*x5*x7^2 - B1*g*cos(x3)*x7;
         x2;
         x6;
         B1*(x2*x8^2 - g*sin(x4));
         B1*x6*x8^2 - B1*g*cos(x4)*x8];

== matlab function BallPlate_FLControl/Feedback linearized 3/Feedback Linearization/Einv_matrix ==
  data: q input; Einv output; dq input
function Einv = fcn(q,dq)

[m_b, r_b, I_b, ~, ~] = Parameters_BP;

x3 = q(3);
x4 = q(4);
x5 = dq(1);
x6 = dq(2);
x7 = dq(3);
x8 = dq(4);

B1 = m_b/(I_b/r_b^2 + m_b);
g = 9.81;

% E = [jacobian(dddy1,x)*g1; jacobian(dddy1,x)*g2;
%      jacobian(dddy2,x)*g1; jacobian(dddy2,x)*g2];

E11 = (2*B1*x5*x7 - B1*g*cos(x3));
E22 = (2*B1*x6*x8 - B1*g*cos(x4));

E = diag([E11, E22]);

Einv = inv(E);

== matlab function BallPlate_FLControl/Feedback linearized 3/Feedback Linearization/Gamma_matrix ==
  data: q input; Gamma output; dq input
function Gamma = fcn(q,dq)

[m_b, r_b, I_b, ~, ~] = Parameters_BP;

x1 = q(1);
x2 = q(2);
x3 = q(3);
x4 = q(4);
x7 = dq(3);
x8 = dq(4);

B1 = m_b/(I_b/r_b^2 + m_b);
g = 9.81;

% Gamma = jacobian(dddy1,x)*f1;
%         jacobian(dddy2,x)*f1];

Gamma1 = B1^2*x7^2*(x1*x7^2 - g*sin(x3)) + B1*g*x7^2*sin(x3);
Gamma2 = B1^2*x8^2*(x2*x8^2 - g*sin(x4)) + B1*g*x8^2*sin(x4);

Gamma = [Gamma1; Gamma2];

== matlab function BallPlate_FLControl/Feedback linearized 3/Subsystem/Ball and Plate dynamic ==
  data: tau input; ddq output; q input; dq input
function ddq = InvDyn_BP(tau, q, dq)

if size(dq,2) == 3
    dq = dq';
end

tau1 = [0; 0; tau(1); tau(2)];

% B, C, G matrices
[B, C, G] = BCG_BP(q, dq);

% Inverse dynamic
ddq = B\(tau1 - C*dq - G); 

end

== matlab function BallPlate_FLControl/Visualization parsing6/MATLAB Function ==
  data: u input; y output
function y = fcn(u)

y = -u;

== matlab function BallPlate_FLControl/Visualization parsing6/Rotation ==
  data: alpha input; R output; beta input
function R = fcn(alpha, beta)

    Rx = [1 0 0; 0 cos(beta) -sin(beta); 0 sin(beta) cos(beta)];
    Ry = [cos(alpha) 0 sin(alpha); 0 1 0; -sin(alpha) 0 cos(alpha)];

R = Rx*Ry;

== matlab function BallPlate_FLControl/Visualization parsing6/Rotation composition/Rotation ==
  data: alpha input; R output; beta input
function R = fcn(alpha, beta)

    alpha = -alpha;
    beta = -beta;
    Rx = [1 0 0; 0 cos(beta) -sin(beta); 0 sin(beta) cos(beta)];
    Ry = [cos(alpha) 0 sin(alpha); 0 1 0; -sin(alpha) 0 cos(alpha)];

R = Rx*Ry;

== matlab function BallPlate_FLControl/Visualization parsing6/Rotation composition 1/Rotation ==
  data: alpha input; R output; beta input
function R = fcn(alpha, beta)
    
    Rx = [1 0 0; 0 cos(beta) -sin(beta); 0 sin(beta) cos(beta)];
    Ry = [cos(alpha) 0 sin(alpha); 0 1 0; -sin(alpha) 0 cos(alpha)];

R = Rx*Ry;

== matlab function BallPlate_FLControl/Feedback linearized 4/Coordinate transform ==
  data: q input; z output; dq input
function z = fcn(q,dq)

    [m_b, r_b, I_b, ~, ~] = Parameters_BP;

    x1 = q(1);
    x2 = q(2);
    x3 = q(3);
    x4 = q(4);
    x5 = dq(1);
    x6 = dq(2);
    x7 = dq(3);
    x8 = dq(4);

    B1 = m_b/(I_b/r_b^2 + m_b);
    g = 9.81;



    z = [x1;
         x5;
         B1*(x1*x7^2 - g*sin(x3));
         B1*x5*x7^2 - B1*g*cos(x3)*x7;
         x2;
         x6;
         B1*(x2*x8^2 - g*sin(x4));
         B1*x6*x8^2 - B1*g*cos(x4)*x8];

== matlab function BallPlate_FLControl/Feedback linearized 4/Feedback Linearization/Einv_matrix ==
  data: q input; Einv output; dq input
function Einv = fcn(q,dq)

[m_b, r_b, I_b, ~, ~] = Parameters_BP;

x3 = q(3);
x4 = q(4);
x5 = dq(1);
x6 = dq(2);
x7 = dq(3);
x8 = dq(4);

B1 = m_b/(I_b/r_b^2 + m_b);
g = 9.81;

% E = [jacobian(dddy1,x)*g1; jacobian(dddy1,x)*g2;
%      jacobian(dddy2,x)*g1; jacobian(dddy2,x)*g2];

E11 = (2*B1*x5*x7 - B1*g*cos(x3));
E22 = (2*B1*x6*x8 - B1*g*cos(x4));

E = diag([E11, E22]);

Einv = inv(E);

== matlab function BallPlate_FLControl/Feedback linearized 4/Feedback Linearization/Gamma_matrix ==
  data: q input; Gamma output; dq input
function Gamma = fcn(q,dq)

[m_b, r_b, I_b, ~, ~] = Parameters_BP;

x1 = q(1);
x2 = q(2);
x3 = q(3);
x4 = q(4);
x7 = dq(3);
x8 = dq(4);

B1 = m_b/(I_b/r_b^2 + m_b);
g = 9.81;

% Gamma = jacobian(dddy1,x)*f1;
%         jacobian(dddy2,x)*f1];

Gamma1 = B1^2*x7^2*(x1*x7^2 - g*sin(x3)) + B1*g*x7^2*sin(x3);
Gamma2 = B1^2*x8^2*(x2*x8^2 - g*sin(x4)) + B1*g*x8^2*sin(x4);

Gamma = [Gamma1; Gamma2];

== matlab function BallPlate_FLControl/Feedback linearized 4/Subsystem/Ball and Plate dynamic ==
  data: tau input; ddq output; q input; dq input
function ddq = InvDyn_BP(tau, q, dq)

if size(dq,2) == 3
    dq = dq';
end

tau1 = [0; 0; tau(1); tau(2)];

% B, C, G matrices
[B, C, G] = BCG_BP(q, dq);

% Inverse dynamic
ddq = B\(tau1 - C*dq - G); 

end

== matlab function BallPlate_FLControl/Feedback linearized 5/Coordinate transform ==
  data: q input; z output; dq input
function z = fcn(q,dq)

    [m_b, r_b, I_b, ~, ~] = Parameters_BP;

    x1 = q(1);
    x2 = q(2);
    x3 = q(3);
    x4 = q(4);
    x5 = dq(1);
    x6 = dq(2);
    x7 = dq(3);
    x8 = dq(4);

    B1 = m_b/(I_b/r_b^2 + m_b);
    g = 9.81;



    z = [x1;
         x5;
         B1*(x1*x7^2 - g*sin(x3));
         B1*x5*x7^2 - B1*g*cos(x3)*x7;
         x2;
         x6;
         B1*(x2*x8^2 - g*sin(x4));
         B1*x6*x8^2 - B1*g*cos(x4)*x8];

== matlab function BallPlate_FLControl/Feedback linearized 5/Feedback Linearization/Einv_matrix ==
  data: q input; Einv output; dq input
function Einv = fcn(q,dq)

[m_b, r_b, I_b, ~, ~] = Parameters_BP;

x3 = q(3);
x4 = q(4);
x5 = dq(1);
x6 = dq(2);
x7 = dq(3);
x8 = dq(4);

B1 = m_b/(I_b/r_b^2 + m_b);
g = 9.81;

% E = [jacobian(dddy1,x)*g1; jacobian(dddy1,x)*g2;
%      jacobian(dddy2,x)*g1; jacobian(dddy2,x)*g2];

E11 = (2*B1*x5*x7 - B1*g*cos(x3));
E22 = (2*B1*x6*x8 - B1*g*cos(x4));

E = diag([E11, E22]);

Einv = inv(E);

== matlab function BallPlate_FLControl/Feedback linearized 5/Feedback Linearization/Gamma_matrix ==
  data: q input; Gamma output; dq input
function Gamma = fcn(q,dq)

[m_b, r_b, I_b, ~, ~] = Parameters_BP;

x1 = q(1);
x2 = q(2);
x3 = q(3);
x4 = q(4);
x7 = dq(3);
x8 = dq(4);

B1 = m_b/(I_b/r_b^2 + m_b);
g = 9.81;

% Gamma = jacobian(dddy1,x)*f1;
%         jacobian(dddy2,x)*f1];

Gamma1 = B1^2*x7^2*(x1*x7^2 - g*sin(x3)) + B1*g*x7^2*sin(x3);
Gamma2 = B1^2*x8^2*(x2*x8^2 - g*sin(x4)) + B1*g*x8^2*sin(x4);

Gamma = [Gamma1; Gamma2];

== matlab function BallPlate_FLControl/Feedback linearized 5/Subsystem/Ball and Plate dynamic ==
  data: tau input; ddq output; q input; dq input
function ddq = InvDyn_BP(tau, q, dq)

if size(dq,2) == 3
    dq = dq';
end

tau1 = [0; 0; tau(1); tau(2)];

% B, C, G matrices
[B, C, G] = BCG_BP(q, dq);

% Inverse dynamic
ddq = B\(tau1 - C*dq - G); 

end

== matlab function BallPlate_FLControl/Visualization parsing7/MATLAB Function ==
  data: u input; y output
function y = fcn(u)

y = -u;

== matlab function BallPlate_FLControl/Visualization parsing7/Rotation ==
  data: alpha input; R output; beta input
function R = fcn(alpha, beta)

    Rx = [1 0 0; 0 cos(beta) -sin(beta); 0 sin(beta) cos(beta)];
    Ry = [cos(alpha) 0 sin(alpha); 0 1 0; -sin(alpha) 0 cos(alpha)];

R = Rx*Ry;

== matlab function BallPlate_FLControl/Visualization parsing7/Rotation composition/Rotation ==
  data: alpha input; R output; beta input
function R = fcn(alpha, beta)

    alpha = -alpha;
    beta = -beta;
    Rx = [1 0 0; 0 cos(beta) -sin(beta); 0 sin(beta) cos(beta)];
    Ry = [cos(alpha) 0 sin(alpha); 0 1 0; -sin(alpha) 0 cos(alpha)];

R = Rx*Ry;

== matlab function BallPlate_FLControl/Visualization parsing7/Rotation composition 1/Rotation ==
  data: alpha input; R output; beta input
function R = fcn(alpha, beta)
    
    Rx = [1 0 0; 0 cos(beta) -sin(beta); 0 sin(beta) cos(beta)];
    Ry = [cos(alpha) 0 sin(alpha); 0 1 0; -sin(alpha) 0 cos(alpha)];

R = Rx*Ry;
